simulink model "Autotrans_shift"  (R2022b)
settings: Solver=VariableStepAuto  StartTime=0.0  StopTime=50.0  RelTol=0.001
model workspace (MATLAB code in the model file):
  | load sldemo_autotrans_data; %load initial conditions and other necessary data
undefined symbols (not defined in the file or in its folder): converter_data, downtab, emap, Hecate_param1, Hecate_param2, Hecate_param3, Hecate_param4, Iei, uptab, vehicledata
settings Model: DataTypeOverride=Off  MinMaxOverflowLogging=ForceOff  SimulationMode=accelerator  LastModifiedBy=fedformi_new
settings SolverCC: ConsecutiveZCsStepRelTol=2.8421709430404e-13
settings DataIOCC: SaveFormat=Array
settings OptimizationCC: BlockReduction=off  BooleanDataType=off
settings DebuggingCC: SaveWithParameterizedLinksMsg=none  UnderspecifiedInitializationDetection=Classic  MergeDetectMultiDrivingBlocksExec=none  SignalResolutionControl=TryResolveAllWithWarning
settings HardwareCC: TargetUnknown=on
settings ModelReferenceCC: PropagateSignalLabelsOutOfModel=off
settings ConfigComp: DVTestSuiteOptimization=Auto  DVDetectOutOfBounds=on  DVModelReferenceHarness=on  DVHarnessSource=Signal Editor

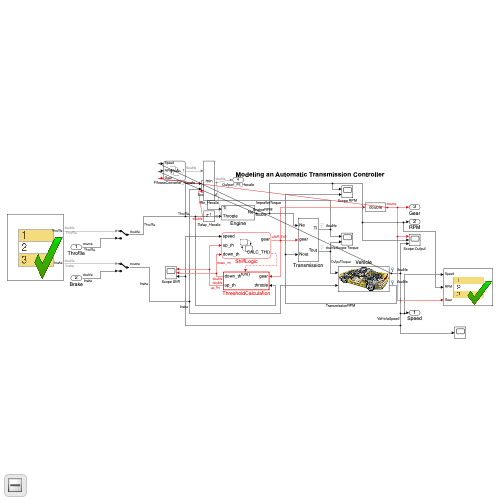
[thumbnail: Simulink's stored preview of the top-level diagram]
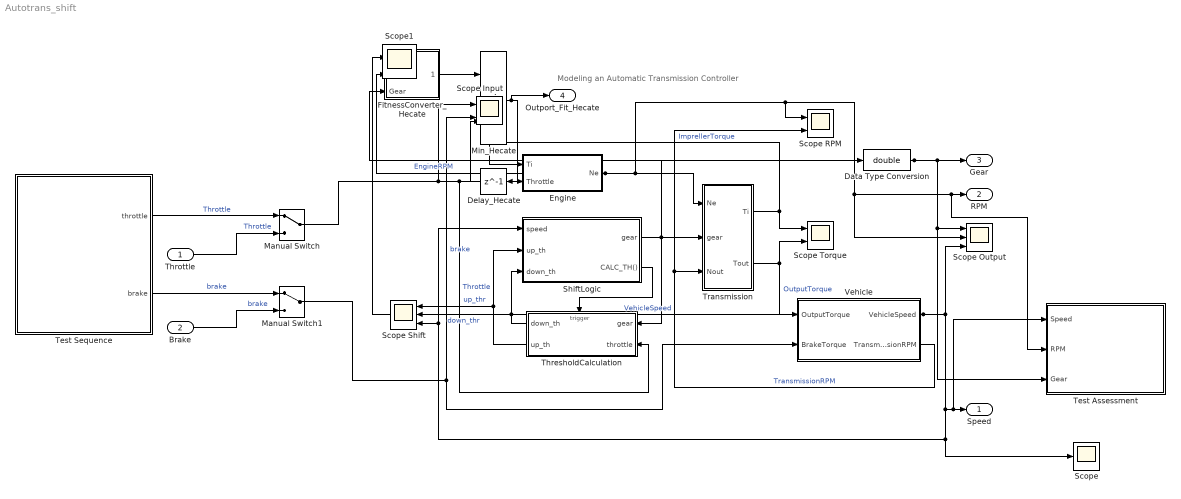
== system Autotrans_shift ==
  note: Modeling an Automatic Transmission Controller
  Throttle : Inport  Interpolate=off
  Brake : Inport  Port=2  Interpolate=off
  Data Type Conversion : DataTypeConversion  OutDataTypeStr=double  SaturateOnIntegerOverflow=off  RndMeth=Floor
  Delay_Hecate : Delay  DelayLength=1  InitialCondition=Inf
  Engine : Subsystem
  FitnessConverter_Hecate : Stateflow chart  TreatAsAtomicUnit=on
  Manual Switch : ManualSwitch
  Manual Switch1 : ManualSwitch
  Min_Hecate : MinMax  Inputs=2
  Scope : Scope
  Scope Input : Scope  NumInputPorts=2
  Scope Output : Scope  NumInputPorts=3
  Scope RPM : Scope  NumInputPorts=2
  Scope Shift : Scope  NumInputPorts=3
  Scope Torque : Scope  NumInputPorts=2
  ShiftLogic : Stateflow chart  TreatAsAtomicUnit=on
  Test Assessment : Test Sequence  TreatAsAtomicUnit=on
  Test Sequence : Test Sequence  TreatAsAtomicUnit=on
  ThresholdCalculation : Subsystem  TreatAsAtomicUnit=on
  Transmission : Subsystem
  Vehicle : Subsystem  mask(vehicle model){Rfd=vehicledata(1), rload0=vehicledata(2), rload2=vehicledata(3), Rw=vehicledata(4), Iv=vehicledata(5), N20=vehicledata(6)/vehicledata(4)*vehicledata(1)}
      mask prompts: Rfd "final drive ratio"; rload0 "drag friction at wheels"; rload2 "aerodynamic drag"; Rw "wheel radius"; Iv "vehicle inertia"; N20 "initial transmission output speed"
      mask help: vehicle dynamics: torque input from trans., outputs are input speed (transmission output) and vehicle speed
      mask Display: image(imread([matlabroot,'/toolbox/simulink/simdemos/automotive/html/NSX_3Colors.jpg']))
  Speed : Outport  VectorParamsAs1DForOutWhenUnconnected=off
  RPM : Outport  Port=2  VectorParamsAs1DForOutWhenUnconnected=off
  Gear : Outport  Port=3  VectorParamsAs1DForOutWhenUnconnected=off
  Outport_Fit_Hecate : Outport  Port=4
  Scope1 : Scope
  wires:
  Transmission/1(Ti) -> Engine/1(Ti), Scope Torque/1  "ImprellerTorque"
  Engine/1(Ne) -> Transmission/1(Ne), Scope RPM/1, Test Assessment/2(RPM), RPM/1, Scope Output/2, FitnessConverter_Hecate/2(RPM)  "EngineRPM"
  Vehicle/2(TransmissionRPM) -> Transmission/3(Nout), Scope RPM/2  "TransmissionRPM"
  ThresholdCalculation/1(down_th) -> Scope Shift/2, ShiftLogic/3(down_th)  "down_thr"
  ThresholdCalculation/2(up_th) -> ShiftLogic/2(up_th), Scope Shift/1  "up_thr"
  ShiftLogic/1(gear) -> Transmission/2(gear), ThresholdCalculation/1(gear), Data Type Conversion/1
  ShiftLogic/2(CALC_TH()) -> ThresholdCalculation/Trigger
  Vehicle/1(VehicleSpeed) -> Scope/1, Scope Shift/3, ShiftLogic/1(speed), Test Assessment/1(Speed), Speed/1, Scope Output/3, FitnessConverter_Hecate/1(Speed)  "VehicleSpeed"
  Manual Switch/1 -> Engine/2(Throttle), ThresholdCalculation/2(throttle), Scope Input/1  "Throttle"
  Transmission/2(Tout) -> Vehicle/1(OutputTorque), Scope Torque/2  "OutputTorque"
  Manual Switch1/1 -> Vehicle/2(BrakeTorque), Scope Input/2  "brake"
  Test Sequence/1(throttle) -> Manual Switch/1  "Throttle"
  Test Sequence/2(brake) -> Manual Switch1/1  "brake"
  Data Type Conversion/1 -> Scope Output/1, Test Assessment/3(Gear), Gear/1, FitnessConverter_Hecate/3(Gear)
  Throttle/1 -> Manual Switch/2  "Throttle"
  Brake/1 -> Manual Switch1/2  "brake"
  FitnessConverter_Hecate/1(fitness_1) -> Min_Hecate/1
  Min_Hecate/1 -> Delay_Hecate/1, Outport_Fit_Hecate/1
  Delay_Hecate/1 -> Min_Hecate/2

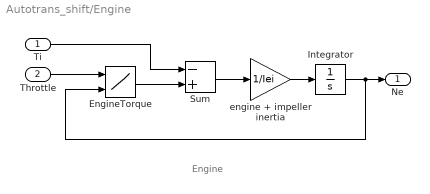
== system Autotrans_shift/Engine ==
  note: Engine
  Ti : Inport
  Throttle : Inport  Port=2
  EngineTorque : Lookup2D  RowIndex=thvec  ColumnIndex=nevec  Table=emap  SaturateOnIntegerOverflow=off
  Integrator : Integrator  InitialCondition=1000  LimitOutput=on  UpperSaturationLimit=6000  LowerSaturationLimit=600  ZeroCross=off
  Sum : Sum  Inputs=-+  InputSameDT=on  SaturateOnIntegerOverflow=on  OutDataTypeStr=Inherit: Same as first input
  engine + impeller inertia : Gain  Gain=1/Iei  SaturateOnIntegerOverflow=on  OutDataTypeStr=Inherit: Same as input  ParamDataTypeStr=Inherit: Same as input
  Ne : Outport  InitialOutput=0  VectorParamsAs1DForOutWhenUnconnected=off
  wires:
  Ti/1 -> Sum/1
  Throttle/1 -> EngineTorque/1
  Integrator/1 -> EngineTorque/2, Ne/1
  Sum/1 -> engine + impeller inertia/1
  engine + impeller inertia/1 -> Integrator/1
  EngineTorque/1 -> Sum/2

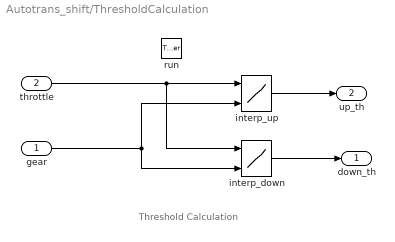
== system Autotrans_shift/ThresholdCalculation ==
  note: Threshold Calculation
  gear : Inport
  throttle : Inport  Port=2
  run : TriggerPort  TriggerType=function-call  VariantControl=(inherit)  ZeroCross=off
  interp_down : Lookup2D  RowIndex=downth  ColumnIndex=[1:4]  Table=downtab  OutDataTypeStr=double  SaturateOnIntegerOverflow=off  InputSameDT=off
      settings: LockScale=on
  interp_up : Lookup2D  RowIndex=upth  ColumnIndex=[1:4]  Table=uptab  OutDataTypeStr=double  SaturateOnIntegerOverflow=off  InputSameDT=off
      settings: LockScale=on
  down_th : Outport  VectorParamsAs1DForOutWhenUnconnected=off
  up_th : Outport  Port=2  VectorParamsAs1DForOutWhenUnconnected=off
  wires:
  interp_up/1 -> up_th/1
  interp_down/1 -> down_th/1
  throttle/1 -> interp_up/1, interp_down/1
  gear/1 -> interp_up/2, interp_down/2

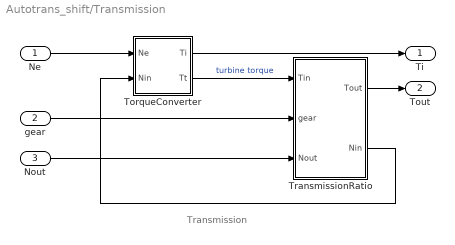
== system Autotrans_shift/Transmission ==
  note: Transmission
  Ne : Inport
  gear : Inport  Port=2
  Nout : Inport  Port=3
  TorqueConverter : Subsystem  mask(torque converter){speedratio=converter_data(:,1), Kfactor=converter_data(:,2), Torkratio=converter_data(:,3)}
      mask prompts: speedratio "speed ratio"; Kfactor "K factor"; Torkratio "torque ratio"
      mask help: torque converter
      mask Help: Torque converter input and output torques are computed as a function of the input and output speeds
      mask Display: plot([cos([90:10:450]*pi/180),.63*cos([90:10:450]*pi/180),.63*cos([90:10:240]*pi/180),cos([240:10:300]*pi/180),.63*cos([300]*pi/180)],[sin([90:10:450]*pi/180),.63*sin([90:10:450]*pi/180)+.1,.63*sin([90:10:240]*pi/180)+.1,sin([240:10:300]*pi/180),.63*sin([300]*pi/180)+.1])
  TransmissionRatio : Subsystem
  Ti : Outport  InitialOutput=0  VectorParamsAs1DForOutWhenUnconnected=off
  Tout : Outport  Port=2  InitialOutput=0  VectorParamsAs1DForOutWhenUnconnected=off
  wires:
  TransmissionRatio/1(Tout) -> Tout/1
  TorqueConverter/1(Ti) -> Ti/1
  Nout/1 -> TransmissionRatio/3(Nout)
  gear/1 -> TransmissionRatio/2(gear)
  Ne/1 -> TorqueConverter/1(Ne)
  TransmissionRatio/2(Nin) -> TorqueConverter/2(Nin)
  TorqueConverter/2(Tt) -> TransmissionRatio/1(Tin)  "turbine torque"

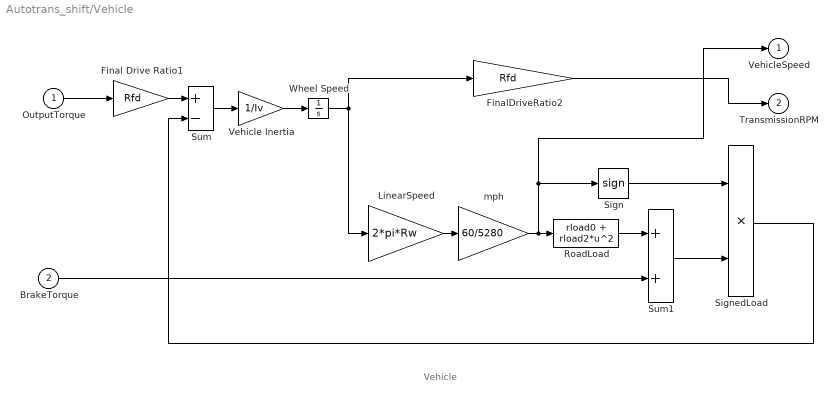
== system Autotrans_shift/Vehicle ==
  note: Vehicle
  OutputTorque : Inport
  BrakeTorque : Inport  Port=2
  Final Drive Ratio1 : Gain  Gain=Rfd  SaturateOnIntegerOverflow=on  OutDataTypeStr=Inherit: Same as input  ParamDataTypeStr=Inherit: Same as input
  FinalDriveRatio2 : Gain  Gain=Rfd  SaturateOnIntegerOverflow=on  OutDataTypeStr=Inherit: Same as input  ParamDataTypeStr=Inherit: Same as input
  LinearSpeed : Gain  Gain=2*pi*Rw  SaturateOnIntegerOverflow=on  OutDataTypeStr=Inherit: Same as input  ParamDataTypeStr=Inherit: Same as input
  RoadLoad : Fcn  Expr=rload0 + rload2*u^2
  Sign : Signum
  SignedLoad : Product  InputSameDT=on  SaturateOnIntegerOverflow=on  OutDataTypeStr=Inherit: Same as first input
  Sum : Sum  Inputs=+-  InputSameDT=on  SaturateOnIntegerOverflow=on  OutDataTypeStr=Inherit: Same as first input
  Sum1 : Sum  InputSameDT=on  SaturateOnIntegerOverflow=on  OutDataTypeStr=Inherit: Same as first input
  Vehicle Inertia : Gain  Gain=1/Iv  SaturateOnIntegerOverflow=on  OutDataTypeStr=Inherit: Same as input  ParamDataTypeStr=Inherit: Same as input
  Wheel Speed : Integrator  InitialCondition=N20/Rfd  ZeroCross=off
  mph : Gain  Gain=60/5280  SaturateOnIntegerOverflow=on  OutDataTypeStr=Inherit: Same as input  ParamDataTypeStr=Inherit: Same as input
  VehicleSpeed : Outport  InitialOutput=0  VectorParamsAs1DForOutWhenUnconnected=off
  TransmissionRPM : Outport  Port=2  InitialOutput=0  VectorParamsAs1DForOutWhenUnconnected=off
  wires:
  FinalDriveRatio2/1 -> TransmissionRPM/1
  BrakeTorque/1 -> Sum1/2
  Sum1/1 -> SignedLoad/2
  RoadLoad/1 -> Sum1/1
  Sign/1 -> SignedLoad/1
  SignedLoad/1 -> Sum/2
  OutputTorque/1 -> Final Drive Ratio1/1
  Vehicle Inertia/1 -> Wheel Speed/1
  Sum/1 -> Vehicle Inertia/1
  mph/1 -> VehicleSpeed/1, Sign/1, RoadLoad/1
  LinearSpeed/1 -> mph/1
  Wheel Speed/1 -> LinearSpeed/1, FinalDriveRatio2/1
  Final Drive Ratio1/1 -> Sum/1

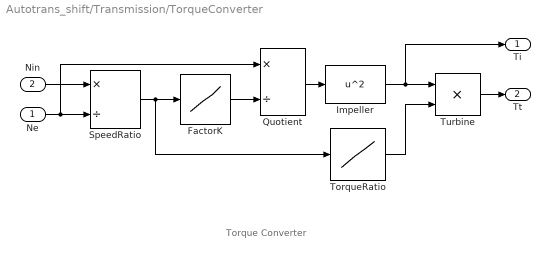
== system Autotrans_shift/Transmission/TorqueConverter ==
  note: Torque Converter
  Ne : Inport
  Nin : Inport  Port=2
  FactorK : Lookup  InputValues=speedratio  Table=Kfactor
  Impeller : Fcn  Expr=u^2
  Quotient : Product  Inputs=*/  InputSameDT=on  SaturateOnIntegerOverflow=on  OutDataTypeStr=Inherit: Same as first input
  SpeedRatio : Product  Inputs=*/  InputSameDT=on  SaturateOnIntegerOverflow=on  OutDataTypeStr=Inherit: Same as first input
  TorqueRatio : Lookup  InputValues=speedratio  Table=Torkratio
  Turbine : Product  InputSameDT=on  SaturateOnIntegerOverflow=on  OutDataTypeStr=Inherit: Same as first input
  Ti : Outport  InitialOutput=0  VectorParamsAs1DForOutWhenUnconnected=off
  Tt : Outport  Port=2  InitialOutput=0  VectorParamsAs1DForOutWhenUnconnected=off
  wires:
  TorqueRatio/1 -> Turbine/2
  Quotient/1 -> Impeller/1
  FactorK/1 -> Quotient/2
  SpeedRatio/1 -> TorqueRatio/1, FactorK/1
  Impeller/1 -> Turbine/1, Ti/1
  Turbine/1 -> Tt/1
  Ne/1 -> SpeedRatio/2, Quotient/1
  Nin/1 -> SpeedRatio/1

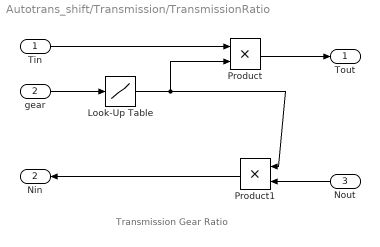
== system Autotrans_shift/Transmission/TransmissionRatio ==
  note: Transmission Gear Ratio
  Tin : Inport
  gear : Inport  Port=2
  Nout : Inport  Port=3
  Look-Up Table : Lookup  InputValues=[1 2 3 4]  Table=[2.393 1.450 1.000 0.677]  OutDataTypeStr=double  LockScale=on
  Product : Product  InputSameDT=on  SaturateOnIntegerOverflow=on  OutDataTypeStr=Inherit: Same as first input
  Product1 : Product  InputSameDT=on  SaturateOnIntegerOverflow=on  OutDataTypeStr=Inherit: Same as first input
  Tout : Outport  InitialOutput=0  VectorParamsAs1DForOutWhenUnconnected=off
  Nin : Outport  Port=2  InitialOutput=0  VectorParamsAs1DForOutWhenUnconnected=off
  wires:
  Look-Up Table/1 -> Product1/1, Product/2
  Nout/1 -> Product1/2
  Product1/1 -> Nin/1
  Product/1 -> Tout/1
  Tin/1 -> Product/1
  gear/1 -> Look-Up Table/1

== stateflow chart Autotrans_shift/FitnessConverter_Hecate ==
  state step_1
    fitness_1 = Inf;
    state step_1_1
      fitness_1 = 120-(Speed);
    state step_1_2
      fitness_1 = Inf;
    (default) -> (junction 4)
    step_1_2 -> (junction 4) : [(((t>=0) && (t<=20)))]
    (junction 4) -> step_1_1 [order 1] : [((t>=0) && (t<=20))]
    (junction 4) -> step_1_2 [order 2] : []
    step_1_1 -> (junction 4) : [~(((t>=0) && (t<=20)))]
  (default) -> step_1
  data: Speed input; RPM input; Gear input; fitness_1 output

== stateflow chart Autotrans_shift/Test Sequence ==
  state step_1
    throttle = Hecate_param1;
    brake=Hecate_param2;
  state step_2
    throttle =Hecate_param3;
    brake = Hecate_param4;
  (default) -> step_1
  step_1 -> step_2 : [
      | et > 10
      | ]
  data: throttle output; brake output; Hecate_param4 parameter; Hecate_param1 parameter; Hecate_param2 parameter; Hecate_param3 parameter

== stateflow chart Autotrans_shift/ShiftLogic ==
  settings: updateMethod=DISCRETE  sampleTime=0.04
  state gear_state [parallel]
    settings: executionOrder=1
    state fourth
      entry:
      gear = 4;
    state third
      entry:
      gear = 3;
    state second
      entry:
      gear = 2;
    state first
      entry:
      gear = 1;
    (default) -> first
    second -> third [order 1] : UP
    first -> second : UP
    third -> fourth [order 1] : UP
    second -> first [order 2] : DOWN
    fourth -> third : DOWN
    third -> second [order 2] : DOWN
  state selection_state [parallel]
    during: CALC_TH;
    settings: executionOrder=2
    state steady_state
    state upshifting
    state downshifting
    (default) -> steady_state
    steady_state -> upshifting [order 1] : [speed > up_th]
    steady_state -> downshifting [order 2] : [speed < down_th]
    downshifting -> steady_state [order 1] : after(TWAIT,tick)
        | [speed <= down_th]
        | {gear_state.DOWN}
    downshifting -> steady_state [order 2] : [speed > down_th]
    upshifting -> steady_state [order 1] : after(TWAIT,tick)
        | [speed >= up_th]
        | {gear_state.UP}
    upshifting -> steady_state [order 2] : [speed < up_th]
  data: speed input double; gear output fixdt(0,8,5) [1..4]; TWAIT parameter fixdt(0,8,6); up_th input double; down_th input double
  events: DOWN local EITHER_EDGE_EVENT; UP local EITHER_EDGE_EVENT; CALC_TH output FUNCTION_CALL_EVENT

== stateflow chart Autotrans_shift/Test Assessment ==
  state AT1
    state step_1
      state step_1_1
        verify(Speed < 120);
        settings: description=|
            | the value of the speed between [0,20]s
            | shall be lower than 120mph
      state step_1_2
      AT1.step_1 -> (junction 405)
      (default) -> (junction 405)
      (junction 405) -> (junction 406) [order 1] : [((t>=0) && (t<=20))
          | ]
      (junction 406) -> AT1.step_1.step_1_1 [order 1] : [~in(AT1.step_1.step_1_1)]
      (junction 406) -> (junction 409) [order 2]
      (junction 725) -> (junction 726)
      (junction 726) -> AT1.step_1.step_1_2 [order 1] : [~in(AT1.step_1.step_1_2)]
      (junction 726) -> (junction 729) [order 2]
      (junction 405) -> (junction 725) [order 2]
    (default) -> AT1.step_1
  state AT2
    state step_1
      state step_1_1
        verify(RPM<4750, 'Message')
      state step_1_2
      (default) -> (junction 433)
      AT2.step_1 -> (junction 433)
      (junction 433) -> (junction 434) [order 1] : [(t>=0 && t<=10)
          | ]
      (junction 434) -> AT2.step_1.step_1_1 [order 1] : [~in(AT2.step_1.step_1_1)]
      (junction 433) -> (junction 733) [order 2]
      (junction 434) -> (junction 437) [order 2]
      (junction 733) -> (junction 734)
      (junction 734) -> AT2.step_1.step_1_2 [order 1] : [~in(AT2.step_1.step_1_2)]
      (junction 734) -> (junction 737) [order 2]
    (default) -> AT2.step_1
  state AT51
    state step_1
    state AT51
      settings: description=Trigger upon changing to gear 1
    state AT51_1
      verify(Gear==1)
    (default) -> AT51.step_1
    AT51.AT51 -> AT51_1 : [
        | (hasChangedTo(Gear,1) && t>=0 && t<=30)
        | ]
    AT51_1 -> AT51.AT51 : [
        | et > 2.5
        | ]
    AT51.step_1 -> AT51.AT51 : [
        | Gear~=1
        | ]
  state AT52
    state AT52
      settings: description=Trigger upon changing to gear 2
    state AT52_1
      verify(Gear==2)
    (default) -> AT52.AT52
    AT52.AT52 -> AT52_1 : [
        | (hasChangedTo(Gear,2) && t>=0 && t<=30)
        | ]
    AT52_1 -> AT52.AT52 : [
        | et > 2.5
        | ]
  state AT53
    state AT53
      settings: description=Trigger upon changing to gear 3
    state AT53_1
      verify(Gear==3)
    (default) -> AT53.AT53
    AT53.AT53 -> AT53_1 : [
        | (hasChangedTo(Gear,3) && t>=0 && t<=30)
        | ]
    AT53_1 -> AT53.AT53 : [
        | et > 2.5
        | ]
  state AT54
    state AT54
      settings: description=Trigger upon changing to gear 4
    state AT54_1
      verify(Gear==4)
    (default) -> AT54.AT54
    AT54.AT54 -> AT54_1 : [
        | (hasChangedTo(Gear,4) && t>=0 && t<=30)
        | ]
    AT54_1 -> AT54.AT54 : [
        | et > 2.5
        | ]
  state AT6a
    state step_1
    state step_2_Inconclusive
    state step_3
    state step_4
    state step_5
      verify(true)
      settings: description=robustness calculation
    state step_6
      verify(false)
    (default) -> AT6a.step_1
    AT6a.step_1 -> (junction 589) [order 2] : [
        | ~(Speed<35)
        | ]
    (junction 589) -> (junction 587)
    AT6a.step_1 -> (junction 593) [order 3] : [
        | t>=4
        | ]
    (junction 593) -> (junction 591)
    AT6a.step_1 -> AT6a.step_2_Inconclusive [order 1] : [
        | ~(RPM<3000)
        | ]
    (junction 608) -> AT6a.step_2_Inconclusive
    (junction 610) -> (junction 608)
    AT6a.step_3 -> AT6a.step_2_Inconclusive [order 1] : [
        | ~(RPM<3000)
        | ]
    (junction 587) -> AT6a.step_3
    AT6a.step_3 -> (junction 758) [order 2] : [
        | t>=30
        | ]
    (junction 758) -> (junction 601)
    AT6a.step_4 -> (junction 610) [order 1] : [
        | ~(RPM<3000)
        | ]
    (junction 591) -> AT6a.step_4
    AT6a.step_4 -> (junction 619) [order 2] : [
        | t>=30
        | ]
    (junction 619) -> (junction 612)
    (junction 601) -> AT6a.step_5
    (junction 612) -> AT6a.step_6
  state AT6b
    state step_1
    state step_2_Inconclusive
    state step_3
    state step_4
    state step_5
      verify(true)
    state step_6
      verify(false)
    AT6b.step_4 -> (junction 658) [order 2] : [
        | t>=30
        | ]
    (default) -> AT6b.step_1
    AT6b.step_1 -> (junction 634) [order 2] : [
        | ~(Speed<50)
        | ]
    (junction 634) -> (junction 632)
    AT6b.step_1 -> (junction 641) [order 3] : [
        | t>=8
        | ]
    (junction 641) -> (junction 639)
    AT6b.step_1 -> AT6b.step_2_Inconclusive [order 1] : [
        | ~(RPM<3000)
        | ]
    (junction 644) -> AT6b.step_2_Inconclusive
    (junction 646) -> (junction 644)
    AT6b.step_3 -> AT6b.step_2_Inconclusive [order 1] : [
        | ~(RPM<3000)
        | ]
    (junction 632) -> AT6b.step_3
    AT6b.step_3 -> (junction 652) [order 2] : [
        | t>=30
        | ]
    (junction 652) -> (junction 650)
    AT6b.step_4 -> (junction 646) [order 1] : [
        | ~(RPM<3000)
        | ]
    (junction 639) -> AT6b.step_4
    (junction 650) -> AT6b.step_5
    (junction 656) -> AT6b.step_6
    (junction 658) -> (junction 656)
  state AT6c
    state step_1
    state step_2_Inconclusive
    state step_3
    state step_4
    state step_5
      verify(true)
    state step_6
      verify(false)
    AT6c.step_4 -> (junction 698) [order 2] : [
        | t>=30
        | ]
    (default) -> AT6c.step_1
    AT6c.step_1 -> (junction 674) [order 2] : [
        | ~(Speed<65)
        | ]
    (junction 674) -> (junction 672)
    AT6c.step_1 -> (junction 681) [order 3] : [
        | t>=20
        | ]
    (junction 681) -> (junction 679)
    AT6c.step_1 -> AT6c.step_2_Inconclusive [order 1] : [
        | ~(RPM<3000)
        | ]
    (junction 684) -> AT6c.step_2_Inconclusive
    (junction 686) -> (junction 684)
    AT6c.step_3 -> AT6c.step_2_Inconclusive [order 1] : [
        | ~(RPM<3000)
        | ]
    (junction 672) -> AT6c.step_3
    AT6c.step_3 -> (junction 692) [order 2] : [
        | t>=30
        | ]
    (junction 692) -> (junction 690)
    AT6c.step_4 -> (junction 686) [order 1] : [
        | ~(RPM<3000)
        | ]
    (junction 679) -> AT6c.step_4
    (junction 690) -> AT6c.step_5
    (junction 696) -> AT6c.step_6
    (junction 698) -> (junction 696)
  (default) -> AT1 [order 1] : [Active_Scenario_Index == 1]
  (default) -> AT2 [order 2] : [Active_Scenario_Index == 2]
  (default) -> AT51 [order 3] : [Active_Scenario_Index == 3]
  (default) -> AT52 [order 4] : [Active_Scenario_Index == 4]
  (default) -> AT53 [order 5] : [Active_Scenario_Index == 5]
  (default) -> AT54 [order 6] : [Active_Scenario_Index == 6]
  (default) -> AT6a [order 7] : [Active_Scenario_Index == 7]
  (default) -> AT6b [order 8] : [Active_Scenario_Index == 8]
  (default) -> AT6c [order 9] : {assert(Active_Scenario_Index == 9,'The value of Scenario Parameter ''Active_Scenario_Index'' is not valid. Use the index of the scenario to specify it.')}
  data: Speed input; RPM input; Gear input; Active_Scenario_Index parameter =1
